simulink model "PubIfDecisionTOS_MDL"  (R2020b)
settings: configuration reference "DspaceConfig" (kept outside this file)
PostLoadFcn:
  | if any(exist('dsrtsu_mdlpostloadfcn', 'file') ~= 0), dsrtsu_mdlpostloadfcn('Execute', bdroot); end
InitFcn:
  | , if any(exist('dsmpb_private', 'file') ~= 0), dsmpb_private('dsmpb_mdlclblib', 'Init', bdroot); end,
undefined symbols (not defined in the file or in its folder): C_TOS_ACCEgoRAxletoFbumplength_m, C_TOS_ACCTargetFront_Flag, C_TOS_AEBJAPedObjDxThre_Val, C_TOS_AEBJAPedObjDyThre_Val, C_TOS_AEBJATargetSize_Val, C_TOS_AEBJAVehObjDxThre_Val, C_TOS_AEBJAVehObjDyThre_Val, C_TOS_AEBJuncPedTargetSize_Val, C_TOS_AEBLatObjDxThre_Val, C_TOS_AEBLatPedDyThre_Val, C_TOS_AEBLatTargetSize_Val, C_TOS_AEBLongTargetInEgoFront_Flag, C_TOS_axAbsGround_Parameter, C_TOS_CameraConfirmedFlag, C_TOS_CNsubjWidth, C_TOS_CurrentLaneCoreMinWidth_Val, C_TOS_CutInProb_Val_Zero, C_TOS_CutOutProb_Val_Zero, C_TOS_D2R_Val, C_TOS_DefaultValueObjectToCenterLine_dy, C_TOS_EgoCarWidth_Val, C_TOS_EgoDxRefPoint_m, C_TOS_EgoRAxletoFbumplength_m, C_TOS_HalfWidthVehicle_Con, C_TOS_HWA_CurrentLaneFlag, C_TOS_HWA_LeftLaneFlag, C_TOS_HWA_MovingDir_Vaild, C_TOS_HWA_MovState_Vaild, C_TOS_HWA_RightLaneFlag, C_TOS_LaneLineCourseErrorFront, C_TOS_LaneLineCourseErrorRear, C_TOS_MotorbikeDefaultWidth_m, C_TOS_NumberOfEffectiveTargets, C_TOS_Obj_Age_Val, C_TOS_Objdx_Constraint_Val, C_TOS_ObjectDefaultWidth_m, C_TOS_ObjInCurrentLane_Val, C_TOS_ObjInCurrentLaneValid, C_TOS_ObjInLeftLaneValid, C_TOS_ObjInRightLaneValid, C_TOS_ObjNotInCurrentLane_Val, C_TOS_ObjNotREElementType, C_TOS_ObjPredictDis_dy_ConstantVal_Zeros, C_TOS_ObjToCenterLine_ConstantVal_Zeros, C_TOS_OFMObjIDInvilad_Val, C_TOS_PIL_LatDisCons_Val_zero, C_TOS_PIL_ObjectCutInFlag_b, C_TOS_PIL_ObjectCutOutFlag_b, C_TOS_PIL_ObjLaneProb_al_Val, C_TOS_PP_ObjFusType_FC_Confirm_b, C_TOS_PP_ObjFusType_FC_FR_Confirm_b, C_TOS_PP_ObjFusType_FR_Confirm_b, C_TOS_RE_80BoolDefault_Val, C_TOS_RE_80Single181Default_Val, C_TOS_RE_80Single255Default_Val, C_TOS_RE_80Uint8Default_Val, C_TOS_RE_D2R, C_TOS_RE_D_180_Val, C_TOS_RE_InvalidObjectID_Val, C_TOS_RE_InvalidTargetChainDir_Val ... (+142)
libraries: simulink x1650, TOS_LIB x361, canfdmsglib x14
(part 24 of 69)

== system PubIfDecisionTOS_MDL/TOS_20201112/TOS_2012080320/PIL_1029/ObjCutInOut_Prob/ObjectCutOut/CutOutProb_Calculate/CutOutProb_Calculate/CutOutPredictDis_dy ==
  note: dx 修正vyc的 cut out 预测时间
  note: vyc的 cut out 基础预测时间
  ObjectToCenterLine_dy_Filt : Inport  OutDataTypeStr=single
  ObjectToCenterLine_dy : Inport  Port=2  OutDataTypeStr=single
  ObjectType : Inport  Port=3
  Object_DX : Inport  Port=4
  PP_ObjectToCenterLine_vyc : Inport  Port=5
  Object_VY : Inport  Port=6
  CutOutPredictTime : Subsystem
  CutOutPredictTime_Constraint1 : Subsystem
  CutOutPredictTime_Constraint2 : Subsystem
  PIL_CutOutPredictTime_ObserVale : Outport  OutDataTypeStr=single
  PIL_CutOutPredictTime_dxConstraint_ObserVale : Outport  Port=2  OutDataTypeStr=single
  CutOutPredictDis_dy : Outport  Port=3  OutDataTypeStr=single
  wires:
  Object_VY/1 -> CutOutPredictTime_Constraint2/4(Object_VY)
  Object_DX/1 -> CutOutPredictTime_Constraint1/2(Object_DX), CutOutPredictTime/5(Object_DX)
  ObjectToCenterLine_dy_Filt/1 -> CutOutPredictTime/1(ObjectToCenterLine_dy_Filt)
  ObjectToCenterLine_dy/1 -> [ObjectToCenterLine_dy], CutOutPredictTime/2(ObjectToCenterLin e_dy)
  CutOutPredictTime/1(CutOutPredictTime) -> [PIL_CutOutPredictTime_ObserVale], CutOutPredictTime_Constraint1/1(CutOutPredictTime)
  CutOutPredictTime_Constraint1/1(CutOutPredictTime_Constraint1) -> CutOutPredictTime_Constraint2/2(PredictTimeConstraint), [PIL_CutOutPredictTime_Constraint_ObserVale]
  PP_ObjectToCenterLine_vyc/1 -> CutOutPredictTime_Constraint2/3(PP_ObjectToCenterLine_vyc), [PP_ObjectToCenterLine_vyc]
  CutOutPredictTime_Constraint2/1(CutOutPredictDis_dy) -> CutOutPredictDis_dy/1
  [ObjectToCenterLine_dy] -> CutOutPredictTime_Constraint2/1(ObjectToCenterLine_dy)
  ObjectType/1 -> CutOutPredictTime/3(ObjectType)
  [PP_ObjectToCenterLine_vyc] -> CutOutPredictTime/4(PP_ObjectToCenterLine_vyc)
  [PIL_CutOutPredictTime_ObserVale] -> PIL_CutOutPredictTime_ObserVale/1
  [PIL_CutOutPredictTime_Constraint_ObserVale] -> PIL_CutOutPredictTime_dxConstraint_ObserVale/1

== system PubIfDecisionTOS_MDL/TOS_20201112/TOS_2012080320/PIL_1029/ObjCutInOut_Prob/ObjectCutOut/CutOutProb_Calculate/CutOutProb_Calculate/CutOutProb ==
  CutOutPredictDis_dy : Inport  OutDataTypeStr=single
  PIL_ObjectToCenterLine_dy_Filt : Inport  Port=2  OutDataTypeStr=single
  Object_Width : Inport  Port=3
  ObjectType : Inport  Port=4
  CutOutObjWidthConstraint : Subsystem
  CutOutProb_Calculation : Subsystem
  PIL_CutOutPredictDis_dy_ObjWidthConstraint_ObserVale : Outport
  CutOutProb : Outport  Port=2
  wires:
  ObjectType/1 -> CutOutObjWidthConstraint/4(ObjectType)
  CutOutProb_Calculation/1(CutOutProb_Calculation) -> CutOutProb/1  "CutInProb_ScopeConstraint"
  CutOutPredictDis_dy/1 -> CutOutObjWidthConstraint/1(CutOutPredictDis_dy)
  PIL_ObjectToCenterLine_dy_Filt/1 -> CutOutObjWidthConstraint/2(PIL_ObjectToCenterLine_dy_Filt), [ObjectToCenterLine_dy]
  Object_Width/1 -> CutOutObjWidthConstraint/3(Object_Width)
  CutOutObjWidthConstraint/1(CutOutPredictDis_dy_ObjWidthConstraint) -> [PIL_CutOutPredictDis_dy_ObjWidthConstraint_ObserVale], CutOutProb_Calculation/1(CutOutPredictDis_dy_ObjWidthConstraint)
  [ObjectToCenterLine_dy] -> CutOutProb_Calculation/2(PIL_ObjectToCenterLine_dy_Filt)
  [PIL_CutOutPredictDis_dy_ObjWidthConstraint_ObserVale] -> PIL_CutOutPredictDis_dy_ObjWidthConstraint_ObserVale/1

== system PubIfDecisionTOS_MDL/TOS_20201112/TOS_2012080320/PIL_1029/ObjCutInOut_Prob/ObjectCutOut/CutOutProb_Calculate/CutOutProb_Calculate/CutOutProb_ScopeConstraint ==
  note: cut out 计算概率值约束
  CutOutProb : Inport  OutDataTypeStr=single
  PIL_ObjectToCenterLine_dy_Filt : Inport  Port=2
  PP_ObjectToCenterLine_vyc : Inport  Port=3  OutDataTypeStr=single
  PP_ObjectToCenterLine_dy : Inport  Port=4  OutDataTypeStr=single
  Object_Width : Inport  Port=5
  ObjectType : Inport  Port=6
  C_CutInProb_Val_Zero : Constant  Value=C_TOS_CutOutProb_Val_Zero  OutDataTypeStr=single
      settings: AttributesFormatString=C_TOS_CutOutProb_Val_Zero = 0
  ObjectCutoutMind : Subsystem
  Switch : Switch  Criteria=u2 ~= 0  OutDataTypeStr=single
  PIL_ObjectCutOutMindFlg_ObserVale : Outport  OutDataTypeStr=boolean
  CutOutProb_ScopeConstraint : Outport  Port=2  OutDataTypeStr=single
  PIL_ObjectCutoutMindFlg1_ObserVale : Outport  Port=3  OutDataTypeStr=boolean
  PIL_ObjectCutoutMindFlg2_ObserVale : Outport  Port=4  OutDataTypeStr=boolean
  PIL_ObjectCutoutMindFlg3_ObserVale : Outport  Port=5  OutDataTypeStr=boolean
  wires:
  ObjectType/1 -> ObjectCutoutMind/5(ObjectType)
  PIL_ObjectToCenterLine_dy_Filt/1 -> ObjectCutoutMind/1(PIL_ObjectToCenterLine_dy_Filt)
  PP_ObjectToCenterLine_vyc/1 -> ObjectCutoutMind/2(PP_ObjectToCenterLine_vyc)
  C_CutInProb_Val_Zero/1 -> Switch/1
  CutOutProb/1 -> Switch/3
  Switch/1 -> CutOutProb_ScopeConstraint/1
  ObjectCutoutMind/1(ObjectCutoutMindFlg) -> [PIL_ObjectCutOutMindFlg_ObserVale], Switch/2
  PP_ObjectToCenterLine_dy/1 -> ObjectCutoutMind/3(PP_ObjectToCenterLine_dy)
  Object_Width/1 -> ObjectCutoutMind/4(Object_Width)
  [PIL_ObjectCutOutMindFlg_ObserVale] -> PIL_ObjectCutOutMindFlg_ObserVale/1
  ObjectCutoutMind/2(ObjectCutoutMindFlg1) -> [ObjectCutoutMindFlg1]
  ObjectCutoutMind/3(ObjectCutoutMindFlg2) -> [ObjectCutoutMindFlg2]
  ObjectCutoutMind/4(ObjectCutoutMindFlg3) -> [ObjectCutoutMindFlg3]
  [ObjectCutoutMindFlg1] -> PIL_ObjectCutoutMindFlg1_ObserVale/1
  [ObjectCutoutMindFlg2] -> PIL_ObjectCutoutMindFlg2_ObserVale/1
  [ObjectCutoutMindFlg3] -> PIL_ObjectCutoutMindFlg3_ObserVale/1

== system PubIfDecisionTOS_MDL/TOS_20201112/TOS_2012080320/PIL_1029/ProbCalculat/ProbCalculat/ObjectProbCalculation/ProbCalculation/LeftLane_LeftPro ==
  PIL_LeftCenterLine_dyc : Inport
  LeftLane_CoreArea_Boundary : Inport  Port=2
  LeftLane_EdgeLeft_Boundary : Inport  Port=3
  Constant1 : Constant  Value=C_TOS_ObjInCurrentLane_Val  OutDataTypeStr=single
      settings: AttributesFormatString=C_TOS_ObjInCurrentLane_Val = 1
  Constant2 : Constant  Value=C_TOS_PIL_LatDisCons_Val_zero
      settings: AttributesFormatString=C_TOS_PIL_LatDisCons_Val_zero = 0
  Constant3 : Constant  Value=C_TOS_ObjNotInCurrentLane_Val  OutDataTypeStr=single
      settings: AttributesFormatString=C_TOS_ObjNotInCurrentLane_Val = 0
  Divide3 : Product  Inputs=*/  OutDataTypeStr=single
  Min : MinMax  Function=max  Inputs=2
  Relational Operator1 : RelationalOperator  Operator=<  OutDataTypeStr=boolean  RndMeth=Nearest
  Relational Operator3 : RelationalOperator  Operator=>  OutDataTypeStr=boolean  RndMeth=Nearest
  Saturation : Saturate  UpperLimit=255  LowerLimit=0.001
  Subtract3 : Sum  Inputs=+-  OutDataTypeStr=single
  Subtract4 : Sum  Inputs=+-  OutDataTypeStr=single
  Switch1 : Switch  Criteria=u2 ~= 0  OutDataTypeStr=single
  Switch2 : Switch  Criteria=u2 ~= 0  OutDataTypeStr=single
  LeftLane_LeftPro : Outport
  wires:
  Divide3/1 -> Switch1/3
  Subtract4/1 -> Saturation/1
  Constant2/1 -> Min/1
  PIL_LeftCenterLine_dyc/1 -> Min/2
  [LeftLane_EdgeLeft_Boundary] -> Subtract4/1, Subtract3/1
  [LeftLane_CoreArea_Boundary] -> Subtract4/2
  Subtract3/1 -> Divide3/1
  [PIL_LeftCenterLine_dyc] -> Subtract3/2
  Switch2/1 -> LeftLane_LeftPro/1
  Switch1/1 -> Switch2/3
  Constant1/1 -> Switch1/1
  Relational Operator1/1 -> Switch1/2
  LeftLane_CoreArea_Boundary/1 -> [LeftLane_CoreArea_Boundary], Relational Operator1/2
  Constant3/1 -> Switch2/1
  Relational Operator3/1 -> Switch2/2
  LeftLane_EdgeLeft_Boundary/1 -> [LeftLane_EdgeLeft_Boundary], Relational Operator3/2
  Min/1 -> Relational Operator1/1, Relational Operator3/1, [PIL_LeftCenterLine_dyc]
  Saturation/1 -> Divide3/2

== system PubIfDecisionTOS_MDL/TOS_20201112/TOS_2012080320/PIL_1029/ProbCalculat/ProbCalculat/ObjectProbCalculation/ProbCalculation/LeftLane_RightPro ==
  PIL_LeftCenterLine_dyc : Inport
  LeftLane_CoreArea_Boundary : Inport  Port=2
  LeftLane_EdgeRight_Boundary : Inport  Port=3
  Abs : Abs
  Constant1 : Constant  Value=C_TOS_ObjInCurrentLane_Val  OutDataTypeStr=single
      settings: AttributesFormatString=C_TOS_ObjInCurrentLane_Val = 1
  Constant2 : Constant  Value=C_TOS_PIL_LatDisCons_Val_zero
      settings: AttributesFormatString=C_TOS_PIL_LatDisCons_Val_zero = 0
  Constant3 : Constant  Value=C_TOS_ObjNotInCurrentLane_Val  OutDataTypeStr=single
      settings: AttributesFormatString=C_TOS_ObjNotInCurrentLane_Val = 0
  Divide3 : Product  Inputs=*/  OutDataTypeStr=single
  Min : MinMax  Inputs=2
  Relational Operator1 : RelationalOperator  Operator=<  OutDataTypeStr=boolean  RndMeth=Nearest
  Relational Operator3 : RelationalOperator  Operator=>  OutDataTypeStr=boolean  RndMeth=Nearest
  Saturation : Saturate  UpperLimit=255  LowerLimit=0.001
  Subtract3 : Sum  Inputs=+-  OutDataTypeStr=single
  Subtract4 : Sum  Inputs=+-  OutDataTypeStr=single
  Switch1 : Switch  Criteria=u2 ~= 0  OutDataTypeStr=single
  Switch2 : Switch  Criteria=u2 ~= 0  OutDataTypeStr=single
  LeftLane_RightPro : Outport
  wires:
  Abs/1 -> [PIL_LeftCenterLine_dyc], Relational Operator3/1, Relational Operator1/1
  Saturation/1 -> Divide3/2
  Min/1 -> Abs/1
  LeftLane_EdgeRight_Boundary/1 -> Relational Operator3/2, [LeftLane_EdgeRight_Boundary]
  Relational Operator3/1 -> Switch2/2
  Constant3/1 -> Switch2/1
  LeftLane_CoreArea_Boundary/1 -> Relational Operator1/2, [LeftLane_CoreArea_Boundary]
  Relational Operator1/1 -> Switch1/2
  Constant1/1 -> Switch1/1
  Switch1/1 -> Switch2/3
  Switch2/1 -> LeftLane_RightPro/1
  [PIL_LeftCenterLine_dyc] -> Subtract3/2
  Subtract3/1 -> Divide3/1
  [LeftLane_CoreArea_Boundary] -> Subtract4/2
  [LeftLane_EdgeRight_Boundary] -> Subtract3/1, Subtract4/1
  PIL_LeftCenterLine_dyc/1 -> Min/2
  Constant2/1 -> Min/1
  Subtract4/1 -> Saturation/1
  Divide3/1 -> Switch1/3

== system PubIfDecisionTOS_MDL/TOS_20201112/TOS_2012080320/PIL_1029/ProbCalculat/ProbCalculat/ObjectProbCalculation/ProbCalculation/RightLane_LeftPro ==
  PIL_RightCenterLine_dyc : Inport
  RightLane_CoreArea_Boundary : Inport  Port=2
  RightLane_EdgeLeft_Boundary : Inport  Port=3
  Constant1 : Constant  Value=C_TOS_ObjInCurrentLane_Val  OutDataTypeStr=single
      settings: AttributesFormatString=C_TOS_ObjInCurrentLane_Val = 1
  Constant2 : Constant  Value=C_TOS_PIL_LatDisCons_Val_zero
      settings: AttributesFormatString=C_TOS_PIL_LatDisCons_Val_zero = 0
  Constant3 : Constant  Value=C_TOS_ObjNotInCurrentLane_Val  OutDataTypeStr=single
      settings: AttributesFormatString=C_TOS_ObjNotInCurrentLane_Val = 0
  Divide3 : Product  Inputs=*/  OutDataTypeStr=single
  Min : MinMax  Function=max  Inputs=2
  Relational Operator1 : RelationalOperator  Operator=<  OutDataTypeStr=boolean  RndMeth=Nearest
  Relational Operator3 : RelationalOperator  Operator=>  OutDataTypeStr=boolean  RndMeth=Nearest
  Saturation : Saturate  UpperLimit=255  LowerLimit=0.001
  Subtract3 : Sum  Inputs=+-  OutDataTypeStr=single
  Subtract4 : Sum  Inputs=+-  OutDataTypeStr=single
  Switch1 : Switch  Criteria=u2 ~= 0  OutDataTypeStr=single
  Switch2 : Switch  Criteria=u2 ~= 0  OutDataTypeStr=single
  RightLane_LeftPro : Outport
  wires:
  Saturation/1 -> Divide3/2
  Min/1 -> [PIL_RightCenterLine_dyc], Relational Operator3/1, Relational Operator1/1
  RightLane_EdgeLeft_Boundary/1 -> Relational Operator3/2, [RightLane_EdgeLeft_Boundary]
  Relational Operator3/1 -> Switch2/2
  Constant3/1 -> Switch2/1
  RightLane_CoreArea_Boundary/1 -> Relational Operator1/2, [RightLane_CoreArea_Boundary]
  Relational Operator1/1 -> Switch1/2
  Constant1/1 -> Switch1/1
  Switch1/1 -> Switch2/3
  Switch2/1 -> RightLane_LeftPro/1
  [PIL_RightCenterLine_dyc] -> Subtract3/2
  Subtract3/1 -> Divide3/1
  [RightLane_CoreArea_Boundary] -> Subtract4/2
  [RightLane_EdgeLeft_Boundary] -> Subtract3/1, Subtract4/1
  PIL_RightCenterLine_dyc/1 -> Min/2
  Constant2/1 -> Min/1
  Subtract4/1 -> Saturation/1
  Divide3/1 -> Switch1/3

== system PubIfDecisionTOS_MDL/TOS_20201112/TOS_2012080320/PIL_1029/ProbCalculat/ProbCalculat/ObjectProbCalculation/ProbCalculation/RightLane_RightPro ==
  PIL_RightCenterLine_dyc : Inport
  RightLane_CoreArea_Boundary : Inport  Port=2
  RightLane_EdgeRight_Boundary : Inport  Port=3
  Abs : Abs
  Constant1 : Constant  Value=C_TOS_ObjInCurrentLane_Val  OutDataTypeStr=single
      settings: AttributesFormatString=C_TOS_ObjInCurrentLane_Val = 1
  Constant2 : Constant  Value=C_TOS_PIL_LatDisCons_Val_zero
      settings: AttributesFormatString=C_TOS_PIL_LatDisCons_Val_zero = 0
  Constant3 : Constant  Value=C_TOS_ObjNotInCurrentLane_Val  OutDataTypeStr=single
      settings: AttributesFormatString=C_TOS_ObjNotInCurrentLane_Val = 0
  Divide3 : Product  Inputs=*/  OutDataTypeStr=single
  Min : MinMax  Inputs=2
  Relational Operator1 : RelationalOperator  Operator=<  OutDataTypeStr=boolean  RndMeth=Nearest
  Relational Operator3 : RelationalOperator  Operator=>  OutDataTypeStr=boolean  RndMeth=Nearest
  Saturation : Saturate  UpperLimit=255  LowerLimit=0.001
  Subtract3 : Sum  Inputs=+-  OutDataTypeStr=single
  Subtract4 : Sum  Inputs=+-  OutDataTypeStr=single
  Switch1 : Switch  Criteria=u2 ~= 0  OutDataTypeStr=single
  Switch2 : Switch  Criteria=u2 ~= 0  OutDataTypeStr=single
  RightLane_RightPro : Outport
  wires:
  Abs/1 -> Relational Operator1/1, Relational Operator3/1, [PIL_RightCenterLine_dyc]
  Divide3/1 -> Switch1/3
  Subtract4/1 -> Saturation/1
  Constant2/1 -> Min/1
  PIL_RightCenterLine_dyc/1 -> Min/2
  [RightLane_EdgeRight_Boundary] -> Subtract4/1, Subtract3/1
  [RightLane_CoreArea_Boundary] -> Subtract4/2
  Subtract3/1 -> Divide3/1
  [PIL_RightCenterLine_dyc] -> Subtract3/2
  Switch2/1 -> RightLane_RightPro/1
  Switch1/1 -> Switch2/3
  Constant1/1 -> Switch1/1
  Relational Operator1/1 -> Switch1/2
  RightLane_CoreArea_Boundary/1 -> [RightLane_CoreArea_Boundary], Relational Operator1/2
  Constant3/1 -> Switch2/1
  Relational Operator3/1 -> Switch2/2
  RightLane_EdgeRight_Boundary/1 -> [RightLane_EdgeRight_Boundary], Relational Operator3/2
  Min/1 -> Abs/1
  Saturation/1 -> Divide3/2

== system PubIfDecisionTOS_MDL/TOS_20201112/TOS_2012080320/PIL_1029/ProbCalculat/ProbCalculat/ObjectProbCalculation/ProbCalculation/SameLane_LeftPro ==
  PIL_SameCenterLine_dyc : Inport
  SameLane_CoreArea_Boundary : Inport  Port=2
  SameLane_EdgeLeft_Boundary : Inport  Port=3
  Constant : Constant  Commented=on  Value=P_TOS_CurrentLaneLeftBasicProb_Val  OutDataTypeStr=single
      settings: AttributesFormatString=P_TOS_CurrentLaneLeftBasicProb_Val = 0.5
  Constant1 : Constant  Value=C_TOS_ObjInCurrentLane_Val  OutDataTypeStr=single
      settings: AttributesFormatString=C_TOS_ObjInCurrentLane_Val = 1
  Constant2 : Constant  Value=C_TOS_PIL_LatDisCons_Val_zero
      settings: AttributesFormatString=C_TOS_PIL_LatDisCons_Val_zero = 0
  Constant3 : Constant  Value=C_TOS_ObjNotInCurrentLane_Val  OutDataTypeStr=single
      settings: AttributesFormatString=C_TOS_ObjNotInCurrentLane_Val = 0
  Divide3 : Product  Inputs=*/  OutDataTypeStr=single
  Min : MinMax  Function=max  Inputs=2
  Relational Operator1 : RelationalOperator  Operator=<  OutDataTypeStr=boolean  RndMeth=Nearest
  Relational Operator3 : RelationalOperator  Operator=>  OutDataTypeStr=boolean  RndMeth=Nearest
  Saturation : Saturate  UpperLimit=255  LowerLimit=0.001
  Subtract3 : Sum  Inputs=+-  OutDataTypeStr=single
  Subtract4 : Sum  Inputs=+-  OutDataTypeStr=single
  Switch1 : Switch  Criteria=u2 ~= 0  OutDataTypeStr=single
  Switch2 : Switch  Criteria=u2 ~= 0  OutDataTypeStr=single
  SameLane_LeftPro : Outport
  wires:
  Saturation/1 -> Divide3/2
  Min/1 -> [PIL_SameCenterLine_dyc], Relational Operator3/1, Relational Operator1/1
  SameLane_EdgeLeft_Boundary/1 -> Relational Operator3/2, [SameLane_EdgeLeft_Boundary]
  Relational Operator3/1 -> Switch2/2
  Constant3/1 -> Switch2/1
  SameLane_CoreArea_Boundary/1 -> Relational Operator1/2, [SameLane_CoreArea_Boundary]
  Relational Operator1/1 -> Switch1/2
  Constant1/1 -> Switch1/1
  Switch1/1 -> Switch2/3
  Switch2/1 -> SameLane_LeftPro/1
  [PIL_SameCenterLine_dyc] -> Subtract3/2
  Subtract3/1 -> Divide3/1
  [SameLane_CoreArea_Boundary] -> Subtract4/2
  [SameLane_EdgeLeft_Boundary] -> Subtract3/1, Subtract4/1
  PIL_SameCenterLine_dyc/1 -> Min/2
  Constant2/1 -> Min/1
  Subtract4/1 -> Saturation/1
  Divide3/1 -> Switch1/3

== system PubIfDecisionTOS_MDL/TOS_20201112/TOS_2012080320/PIL_1029/ProbCalculat/ProbCalculat/ObjectProbCalculation/ProbCalculation/SameLane_RightPro ==
  PIL_SameCenterLine_dyc : Inport
  SameLane_CoreArea_Boundary : Inport  Port=2
  SameLane_EdgeRight_Boundary : Inport  Port=3
  Abs : Abs
  Constant1 : Constant  Value=C_TOS_ObjInCurrentLane_Val  OutDataTypeStr=single
      settings: AttributesFormatString=C_TOS_ObjInCurrentLane_Val = 1
  Constant2 : Constant  Value=C_TOS_PIL_LatDisCons_Val_zero
      settings: AttributesFormatString=C_TOS_PIL_LatDisCons_Val_zero = 0
  Constant3 : Constant  Value=C_TOS_ObjNotInCurrentLane_Val  OutDataTypeStr=single
      settings: AttributesFormatString=C_TOS_ObjNotInCurrentLane_Val = 0
  Constant4 : Constant  Commented=on  Value=P_TOS_CurrentLaneRightBasicProb_Val  OutDataTypeStr=single
      settings: AttributesFormatString=P_TOS_CurrentLaneRightBasicProb_Val = 0.5
  Divide3 : Product  Inputs=*/  OutDataTypeStr=single
  Min : MinMax  Inputs=2
  Relational Operator1 : RelationalOperator  Operator=<  OutDataTypeStr=boolean  RndMeth=Nearest
  Relational Operator3 : RelationalOperator  Operator=>  OutDataTypeStr=boolean  RndMeth=Nearest
  Saturation : Saturate  UpperLimit=255  LowerLimit=0.001
  Subtract3 : Sum  Inputs=+-  OutDataTypeStr=single
  Subtract4 : Sum  Inputs=+-  OutDataTypeStr=single
  Switch1 : Switch  Criteria=u2 ~= 0  OutDataTypeStr=single
  Switch2 : Switch  Criteria=u2 ~= 0  OutDataTypeStr=single
  SameLane_RightPro : Outport
  wires:
  Abs/1 -> Relational Operator1/1, Relational Operator3/1, [PIL_SameCenterLine_dyc]
  Divide3/1 -> Switch1/3
  Subtract4/1 -> Saturation/1
  Constant2/1 -> Min/1
  PIL_SameCenterLine_dyc/1 -> Min/2
  [SameLane_EdgeRight_Boundary] -> Subtract4/1, Subtract3/1
  [SameLane_CoreArea_Boundary] -> Subtract4/2
  Subtract3/1 -> Divide3/1
  [PIL_SameCenterLine_dyc] -> Subtract3/2
  Switch2/1 -> SameLane_RightPro/1
  Switch1/1 -> Switch2/3
  Constant1/1 -> Switch1/1
  Relational Operator1/1 -> Switch1/2
  SameLane_CoreArea_Boundary/1 -> [SameLane_CoreArea_Boundary], Relational Operator1/2
  Constant3/1 -> Switch2/1
  Relational Operator3/1 -> Switch2/2
  SameLane_EdgeRight_Boundary/1 -> [SameLane_EdgeRight_Boundary], Relational Operator3/2
  Min/1 -> Abs/1
  Saturation/1 -> Divide3/2

== system PubIfDecisionTOS_MDL/TOS_20201112/TOS_2012080320/PIL_1029/ProbCalculat/ProbCalculat/Subsystem/EgoVehiclePro/EgoLaneProb ==
  HalfEgoWidth : Inport
  t_dleft_EgoLane : Inport  Port=2
  t_dright_EgoLane : Inport  Port=3
  Add : Sum  Inputs=+-
  Add1 : Sum  Inputs=+-
  Add2 : Sum  Inputs=+-
  Constant : Constant  Value=0  OutDataTypeStr=single
  Constant1 : Constant  OutDataTypeStr=single
  Constant2 : Constant  Value=0  OutDataTypeStr=single
  Constant3 : Constant  OutDataTypeStr=single
  Divide : Product  Inputs=*/
  Divide1 : Product  Inputs=*/
  Gain1 : Gain  Gain=-1
  Gain2 : Gain  Gain=2
  Gain3 : Gain  Gain=-1
  Gain4 : Gain  Gain=2
  Relational Operator1 : RelationalOperator  Operator=<=  OutDataTypeStr=boolean  RndMeth=Nearest
  Relational Operator2 : RelationalOperator  Operator=>  OutDataTypeStr=boolean  RndMeth=Nearest
  Relational Operator3 : RelationalOperator  Operator=<=  OutDataTypeStr=boolean  RndMeth=Nearest
  Relational Operator4 : RelationalOperator  Operator=>  OutDataTypeStr=boolean  RndMeth=Nearest
  Switch{1..4} (4 alike) : Switch  Criteria=u2 > Threshold
  " EgoLaneProb" : Outport
  wires:
  Switch2/1 -> Add2/1  "t_dleftProb"
  t_dleft_EgoLane/1 -> Add/1, Relational Operator2/1, Relational Operator1/1
  Gain1/1 -> Relational Operator1/2, Add/2
  Relational Operator1/1 -> Switch2/2
  Constant/1 -> Switch2/1
  Relational Operator2/1 -> Switch1/2
  Switch1/1 -> Switch2/3
  Constant1/1 -> Switch1/1
  Add/1 -> Divide/1
  Divide/1 -> Switch1/3
  Gain2/1 -> Divide/2
  Gain4/1 -> Divide1/2
  HalfEgoWidth/1 -> Gain2/1, Gain3/1, Relational Operator4/2, Gain4/1, Relational Operator2/2, Gain1/1
  Divide1/1 -> Switch3/3
  Add1/1 -> Divide1/1
  Constant3/1 -> Switch3/1
  Switch3/1 -> Switch4/3
  Relational Operator4/1 -> Switch3/2
  Constant2/1 -> Switch4/1
  Relational Operator3/1 -> Switch4/2
  Gain3/1 -> Add1/2, Relational Operator3/2
  t_dright_EgoLane/1 -> Relational Operator3/1, Relational Operator4/1, Add1/1
  Switch4/1 -> Add2/2  "t_drightProb"
  Add2/1 -> " EgoLaneProb"/1

== system PubIfDecisionTOS_MDL/TOS_20201112/TOS_2012080320/PIL_1029/ProbCalculat/ProbCalculat/Subsystem/EgoVehiclePro/LeftLaneProb ==
  HalfEgoWidth : Inport
  t_dleft_LeftLane : Inport  Port=2
  t_dright_LeftLane : Inport  Port=3
  Add : Sum  Inputs=+-
  Add1 : Sum  Inputs=+-
  Add2 : Sum  Inputs=+-
  Constant : Constant  Value=0  OutDataTypeStr=single
  Constant1 : Constant  OutDataTypeStr=single
  Constant2 : Constant  Value=0  OutDataTypeStr=single
  Constant3 : Constant  OutDataTypeStr=single
  Divide : Product  Inputs=*/  OutDataTypeStr=single
  Divide1 : Product  Inputs=*/  OutDataTypeStr=single
  Gain1 : Gain  Gain=-1
  Gain2 : Gain  Gain=2
  Gain3 : Gain  Gain=-1
  Gain4 : Gain  Gain=2
  Relational Operator1 : RelationalOperator  Operator=<=  OutDataTypeStr=boolean  RndMeth=Nearest
  Relational Operator2 : RelationalOperator  Operator=>  OutDataTypeStr=boolean  RndMeth=Nearest
  Relational Operator3 : RelationalOperator  Operator=<=  OutDataTypeStr=boolean  RndMeth=Nearest
  Relational Operator4 : RelationalOperator  Operator=>  OutDataTypeStr=boolean  RndMeth=Nearest
  Switch{1..4} (4 alike) : Switch  Criteria=u2 > Threshold
  " LeftLaneProb" : Outport
  wires:
  Switch4/1 -> Add2/2  "t_drightProb"
  t_dright_LeftLane/1 -> Add1/1, Relational Operator4/1, Relational Operator3/1
  Gain3/1 -> Relational Operator3/2, Add1/2
  Relational Operator3/1 -> Switch4/2
  Constant2/1 -> Switch4/1
  Relational Operator4/1 -> Switch3/2
  Switch3/1 -> Switch4/3
  Constant3/1 -> Switch3/1
  Add1/1 -> Divide1/1
  Divide1/1 -> Switch3/3
  HalfEgoWidth/1 -> Gain1/1, Relational Operator2/2, Gain4/1, Relational Operator4/2, Gain3/1, Gain2/1
  Gain4/1 -> Divide1/2
  Gain2/1 -> Divide/2
  Divide/1 -> Switch1/3
  Add/1 -> Divide/1
  Constant1/1 -> Switch1/1
  Switch1/1 -> Switch2/3
  Relational Operator2/1 -> Switch1/2
  Constant/1 -> Switch2/1
  Relational Operator1/1 -> Switch2/2
  Gain1/1 -> Add/2, Relational Operator1/2
  t_dleft_LeftLane/1 -> Relational Operator1/1, Relational Operator2/1, Add/1
  Switch2/1 -> Add2/1  "t_dleftProb"
  Add2/1 -> " LeftLaneProb"/1

== system PubIfDecisionTOS_MDL/TOS_20201112/TOS_2012080320/PIL_1029/ProbCalculat/ProbCalculat/Subsystem/EgoVehiclePro/RightLaneProb ==
  HalfEgoWidth : Inport
  t_dleft_RightLane : Inport  Port=2
  t_dright_RightLane : Inport  Port=3
  Add : Sum  Inputs=+-
  Add1 : Sum  Inputs=+-
  Add2 : Sum  Inputs=+-
  Constant : Constant  Value=0  OutDataTypeStr=single
  Constant1 : Constant  OutDataTypeStr=single
  Constant2 : Constant  Value=0  OutDataTypeStr=single
  Constant3 : Constant  OutDataTypeStr=single
  Divide : Product  Inputs=*/
  Divide1 : Product  Inputs=*/
  Gain1 : Gain  Gain=-1
  Gain2 : Gain  Gain=2
  Gain3 : Gain  Gain=-1
  Gain4 : Gain  Gain=2
  Relational Operator1 : RelationalOperator  Operator=<=  OutDataTypeStr=boolean  RndMeth=Nearest
  Relational Operator2 : RelationalOperator  Operator=>  OutDataTypeStr=boolean  RndMeth=Nearest
  Relational Operator3 : RelationalOperator  Operator=<=  OutDataTypeStr=boolean  RndMeth=Nearest
  Relational Operator4 : RelationalOperator  Operator=>  OutDataTypeStr=boolean  RndMeth=Nearest
  Switch{1..4} (4 alike) : Switch  Criteria=u2 > Threshold
  " RightLaneProb" : Outport
  wires:
  t_dleft_RightLane/1 -> Add/1, Relational Operator2/1, Relational Operator1/1
  Gain1/1 -> Relational Operator1/2, Add/2
  Relational Operator1/1 -> Switch2/2
  Constant/1 -> Switch2/1
  Relational Operator2/1 -> Switch1/2
  Switch1/1 -> Switch2/3
  Constant1/1 -> Switch1/1
  Add/1 -> Divide/1
  Divide/1 -> Switch1/3
  Gain2/1 -> Divide/2
  Gain4/1 -> Divide1/2
  HalfEgoWidth/1 -> Gain2/1, Gain3/1, Relational Operator4/2, Gain4/1, Relational Operator2/2, Gain1/1
  Divide1/1 -> Switch3/3
  Add1/1 -> Divide1/1
  Constant3/1 -> Switch3/1
  Switch3/1 -> Switch4/3
  Relational Operator4/1 -> Switch3/2
  Constant2/1 -> Switch4/1
  Relational Operator3/1 -> Switch4/2
  Gain3/1 -> Add1/2, Relational Operator3/2
  t_dright_RightLane/1 -> Relational Operator3/1, Relational Operator4/1, Add1/1
  Add2/1 -> " RightLaneProb"/1
  Switch2/1 -> Add2/1  "t_dleftProb"
  Switch4/1 -> Add2/2  "t_drightProb"

== system PubIfDecisionTOS_MDL/TOS_20201112/TOS_2012080320/PIL_1029/ProbCalculat/ProbCalculat/Subsystem/PIL_EgoVehiclePro/EgoVehicle_EgoLaneProb ==
  EgoCar_CurrentLaneProb : Inport
  Add : Sum  Inputs=++++
  Add1 : Sum  Inputs=++++
  Bus Creator : BusCreator  Inputs=4
  Bus Selector : BusSelector  OutputSignals=Out_Prob1.Count1,Out_Prob2.Count2,Out_Prob3.Count3,Out_Prob4.Count4
  Bus Selector2 : BusSelector  OutputSignals=Out_Prob1.Prob1,Out_Prob2.Prob2,Out_Prob3.Prob3,Out_Prob4.Prob4
  Compare To Constant : simulink/Logic and Bit Operations/Compare To Constant  relop=~=  const=0  OutDataTypeStr=boolean
  Constant1 : Constant  OutDataTypeStr=single
  Data1 : Subsystem
  Data10 : Subsystem
  Data2 : Subsystem
  Data3 : Subsystem
  Data4 : Subsystem
  Data5 : Subsystem
  Data6 : Subsystem
  Data7 : Subsystem
  Data8 : Subsystem
  Data9 : Subsystem
  Delay : Delay  DelayLength=1  InitialCondition=0
  Delay1 : Delay  InitialCondition=0
  Delay2 : Delay  DelayLength=3  InitialCondition=0
  Delay3 : Delay  DelayLength=4  InitialCondition=0
  Delay4 : Delay  DelayLength=5  InitialCondition=0
  Delay5 : Delay  DelayLength=6  InitialCondition=0
  Delay6 : Delay  DelayLength=7  InitialCondition=0
  Delay7 : Delay  DelayLength=8  InitialCondition=0
  Delay8 : Delay  DelayLength=9  InitialCondition=0
  Divide : Product  Inputs=*/
  Switch : Switch  Criteria=u2 > Threshold
  Terminator{,1..5} (6 alike) : Terminator
  EgoCar_CurrentLaneProb_Filt : Outport
  wires:
  Switch/1 -> Divide/2
  Delay5/1 -> Data7/1(Prob)
  Delay3/1 -> Data5/1(Prob)
  Data4/1(Out_Prob4) -> Bus Creator/4
  Delay1/1 -> Data3/1(Prob)
  Delay8/1 -> Data10/1(Prob)
  Data8/1(Out_Prob8) -> Terminator3/1
  Add/1 -> Compare To Constant/1, Switch/1
  Constant1/1 -> Switch/3
  Delay6/1 -> Data8/1(Prob)
  Data10/1(Out_Prob10) -> Terminator5/1
  Compare To Constant/1 -> Switch/2
  Data5/1(Out_Prob5) -> Terminator/1
  Bus Creator/1 -> Bus Selector/1, Bus Selector2/1
  Data2/1(Out_Prob2) -> Bus Creator/2
  Data1/1(Out_Prob1) -> Bus Creator/1
  Data9/1(Out_Prob9) -> Terminator4/1
  Delay7/1 -> Data9/1(Prob)
  Delay4/1 -> Data6/1(Prob)
  Delay/1 -> Data2/1(Prob)
  Data6/1(Out_Prob6) -> Terminator1/1
  Data7/1(Out_Prob7) -> Terminator2/1
  Delay2/1 -> Data4/1(Prob)
  EgoCar_CurrentLaneProb/1 -> Delay1/1, Delay8/1, Delay7/1, Delay6/1, Delay5/1, Delay4/1, Delay3/1, Delay2/1, Delay/1, Data1/1(Prob)
  Add1/1 -> Divide/1
  Data3/1(Out_Prob3) -> Bus Creator/3
  Divide/1 -> EgoCar_CurrentLaneProb_Filt/1
  Bus Selector/1 -> Add/1  "<Count1>"
  Bus Selector/2 -> Add/2  "<Count2>"
  Bus Selector/3 -> Add/3  "<Count3>"
  Bus Selector/4 -> Add/4  "<Count4>"
  Bus Selector2/1 -> Add1/1  "<Prob1>"
  Bus Selector2/2 -> Add1/2  "<Prob2>"
  Bus Selector2/3 -> Add1/3  "<Prob3>"
  Bus Selector2/4 -> Add1/4  "<Prob4>"

== system PubIfDecisionTOS_MDL/TOS_20201112/TOS_2012080320/PIL_1029/ProbCalculat/ProbCalculat/Subsystem/PIL_EgoVehiclePro/EgoVehicle_LeftLaneProb ==
  EgoVehicle_LeftLaneProb : Inport
  Add : Sum  Inputs=++++
  Add1 : Sum  Inputs=++++
  Bus Creator : BusCreator  Inputs=4
  Bus Selector : BusSelector  OutputSignals=Out_Prob1.Count1,Out_Prob2.Count2,Out_Prob3.Count3,Out_Prob4.Count4
  Bus Selector2 : BusSelector  OutputSignals=Out_Prob1.Prob1,Out_Prob2.Prob2,Out_Prob3.Prob3,Out_Prob4.Prob4
  Compare To Constant : simulink/Logic and Bit Operations/Compare To Constant  relop=~=  const=0  OutDataTypeStr=boolean
  Constant1 : Constant  OutDataTypeStr=single
  Data1 : Subsystem
  Data10 : Subsystem
  Data2 : Subsystem
  Data3 : Subsystem
  Data4 : Subsystem
  Data5 : Subsystem
  Data6 : Subsystem
  Data7 : Subsystem
  Data8 : Subsystem
  Data9 : Subsystem
  Delay : Delay  DelayLength=1  InitialCondition=0
  Delay1 : Delay  InitialCondition=0
  Delay2 : Delay  DelayLength=3  InitialCondition=0
  Delay3 : Delay  DelayLength=4  InitialCondition=0
  Delay4 : Delay  DelayLength=5  InitialCondition=0
  Delay5 : Delay  DelayLength=6  InitialCondition=0
  Delay6 : Delay  DelayLength=7  InitialCondition=0
  Delay7 : Delay  DelayLength=8  InitialCondition=0
  Delay8 : Delay  DelayLength=9  InitialCondition=0
  Divide : Product  Inputs=*/
  Switch : Switch  Criteria=u2 > Threshold
  Terminator{,1..5} (6 alike) : Terminator
  EgoVehicle_LeftLaneProb_Filt : Outport
  wires:
  Divide/1 -> EgoVehicle_LeftLaneProb_Filt/1
  Data3/1(Out_Prob3) -> Bus Creator/3
  Add1/1 -> Divide/1
  EgoVehicle_LeftLaneProb/1 -> Data1/1(Prob), Delay/1, Delay2/1, Delay3/1, Delay4/1, Delay5/1, Delay6/1, Delay7/1, Delay8/1, Delay1/1
  Delay2/1 -> Data4/1(Prob)
  Data7/1(Out_Prob7) -> Terminator2/1
  Data6/1(Out_Prob6) -> Terminator1/1
  Delay/1 -> Data2/1(Prob)
  Delay4/1 -> Data6/1(Prob)
  Delay7/1 -> Data9/1(Prob)
  Data9/1(Out_Prob9) -> Terminator4/1
  Data1/1(Out_Prob1) -> Bus Creator/1
  Data2/1(Out_Prob2) -> Bus Creator/2
  Bus Creator/1 -> Bus Selector2/1, Bus Selector/1
  Data5/1(Out_Prob5) -> Terminator/1
  Compare To Constant/1 -> Switch/2
  Data10/1(Out_Prob10) -> Terminator5/1
  Bus Selector/1 -> Add/1  "<Count1>"
  Delay6/1 -> Data8/1(Prob)
  Constant1/1 -> Switch/3
  Add/1 -> Switch/1, Compare To Constant/1
  Data8/1(Out_Prob8) -> Terminator3/1
  Delay8/1 -> Data10/1(Prob)
  Delay1/1 -> Data3/1(Prob)
  Data4/1(Out_Prob4) -> Bus Creator/4
  Delay3/1 -> Data5/1(Prob)
  Delay5/1 -> Data7/1(Prob)
  Switch/1 -> Divide/2
  Bus Selector/2 -> Add/2  "<Count2>"
  Bus Selector/3 -> Add/3  "<Count3>"
  Bus Selector/4 -> Add/4  "<Count4>"
  Bus Selector2/1 -> Add1/1  "<Prob1>"
  Bus Selector2/2 -> Add1/2  "<Prob2>"
  Bus Selector2/3 -> Add1/3  "<Prob3>"
  Bus Selector2/4 -> Add1/4  "<Prob4>"

== system PubIfDecisionTOS_MDL/TOS_20201112/TOS_2012080320/PIL_1029/ProbCalculat/ProbCalculat/Subsystem/PIL_EgoVehiclePro/EgoVehicle_RightLaneProb ==
  EgoVehicle_RightLaneProb : Inport
  Add : Sum  Inputs=++++
  Add1 : Sum  Inputs=++++
  Bus Creator1 : BusCreator  Inputs=4
  Bus Selector : BusSelector  OutputSignals=Out_Prob1.Count1,Out_Prob2.Count2,Out_Prob3.Count3,Out_Prob4.Count4
  Bus Selector2 : BusSelector  OutputSignals=Out_Prob1.Prob1,Out_Prob2.Prob2,Out_Prob3.Prob3,Out_Prob4.Prob4
  Compare To Constant : simulink/Logic and Bit Operations/Compare To Constant  relop=~=  const=0  OutDataTypeStr=boolean
  Constant1 : Constant  OutDataTypeStr=single
  Data1 : Subsystem
  Data10 : Subsystem
  Data2 : Subsystem
  Data3 : Subsystem
  Data4 : Subsystem
  Data5 : Subsystem
  Data6 : Subsystem
  Data7 : Subsystem
  Data8 : Subsystem
  Data9 : Subsystem
  Delay : Delay  DelayLength=1  InitialCondition=0
  Delay1 : Delay  InitialCondition=0
  Delay2 : Delay  DelayLength=3  InitialCondition=0
  Delay3 : Delay  DelayLength=4  InitialCondition=0
  Delay4 : Delay  DelayLength=5  InitialCondition=0
  Delay5 : Delay  DelayLength=6  InitialCondition=0
  Delay6 : Delay  DelayLength=7  InitialCondition=0
  Delay7 : Delay  DelayLength=8  InitialCondition=0
  Delay8 : Delay  DelayLength=9  InitialCondition=0
  Divide : Product  Inputs=*/
  Switch : Switch  Criteria=u2 > Threshold
  Terminator{6..11} (6 alike) : Terminator
  EgoVehicle_RightLaneProb_Filt : Outport
  wires:
  Divide/1 -> EgoVehicle_RightLaneProb_Filt/1
  Data3/1(Out_Prob3) -> Bus Creator1/3
  Add1/1 -> Divide/1
  EgoVehicle_RightLaneProb/1 -> Data1/1(Prob), Delay/1, Delay2/1, Delay3/1, Delay4/1, Delay5/1, Delay6/1, Delay7/1, Delay8/1, Delay1/1
  Delay2/1 -> Data4/1(Prob)
  Data7/1(Out_Prob7) -> Terminator8/1
  Data6/1(Out_Prob6) -> Terminator7/1
  Delay/1 -> Data2/1(Prob)
  Delay4/1 -> Data6/1(Prob)
  Delay7/1 -> Data9/1(Prob)
  Data9/1(Out_Prob9) -> Terminator10/1
  Data1/1(Out_Prob1) -> Bus Creator1/1
  Data2/1(Out_Prob2) -> Bus Creator1/2
  Bus Creator1/1 -> Bus Selector2/1, Bus Selector/1
  Data5/1(Out_Prob5) -> Terminator6/1
  Compare To Constant/1 -> Switch/2
  Data10/1(Out_Prob10) -> Terminator11/1
  Delay6/1 -> Data8/1(Prob)
  Constant1/1 -> Switch/3
  Add/1 -> Switch/1, Compare To Constant/1
  Data8/1(Out_Prob8) -> Terminator9/1
  Delay8/1 -> Data10/1(Prob)
  Delay1/1 -> Data3/1(Prob)
  Data4/1(Out_Prob4) -> Bus Creator1/4
  Delay3/1 -> Data5/1(Prob)
  Delay5/1 -> Data7/1(Prob)
  Switch/1 -> Divide/2
  Bus Selector2/1 -> Add1/1  "<Prob1>"
  Bus Selector2/2 -> Add1/2  "<Prob2>"
  Bus Selector2/3 -> Add1/3  "<Prob3>"
  Bus Selector2/4 -> Add1/4  "<Prob4>"
  Bus Selector/1 -> Add/1  "<Count1>"
  Bus Selector/2 -> Add/2  "<Count2>"
  Bus Selector/3 -> Add/3  "<Count3>"
  Bus Selector/4 -> Add/4  "<Count4>"

== system PubIfDecisionTOS_MDL/TOS_20201112/TOS_2012080320/PP1128/AAT-AdditionalAttributes/PP_CenterLine_Calculat/LaneWidth_80/LaneWidth/PP_LaneWidth ==
  LM_SignalVerification : Inport
  Action Port : ActionPort
  Add : Sum  Inputs=+-  OutDataTypeStr=single
  Add1 : Sum  Inputs=+-  OutDataTypeStr=single
  Add2 : Sum  Inputs=+-  OutDataTypeStr=single
  Bus Selector : BusSelector  OutputSignals=LM_LL_pC0,LM_LR_pC0,LM_RL_pC0,LM_RR_pC0
  Saturation : Saturate  UpperLimit=4.5  LowerLimit=2.0  OutDataTypeStr=single
  Saturation1 : Saturate  UpperLimit=4.5  LowerLimit=2.0  OutDataTypeStr=single
  Saturation2 : Saturate  UpperLimit=4.5  LowerLimit=2.0  OutDataTypeStr=single
  Signal Copy{,1..3} (4 alike) : SignalConversion  OverrideOpt=off
  TOS_PP_LeftLaneWidth : Outport
  TOS_PP_CurrentLaneWidth : Outport  Port=2
  TOS_PP_RightLaneWidth : Outport  Port=3
  wires:
  Bus Selector/1 -> Signal Copy/1  "<LM_LL_pC0>"
  Bus Selector/4 -> Signal Copy3/1  "<LM_RR_pC0>"
  LM_SignalVerification/1 -> Bus Selector/1
  Bus Selector/3 -> Signal Copy2/1  "<LM_RL_pC0>"
  Bus Selector/2 -> Signal Copy1/1  "<LM_LR_pC0>"
  Add/1 -> Saturation/1
  Add2/1 -> Saturation2/1
  Add1/1 -> Saturation1/1
  Signal Copy1/1 -> Add/2, Add1/1  "LM_LR_pC0"
  Signal Copy/1 -> Add/1  "LM_LL_pC0"
  Signal Copy3/1 -> Add2/2  "LM_RR_pC0"
  Signal Copy2/1 -> Add2/1, Add1/2  "LM_RL_pC0"
  Saturation/1 -> TOS_PP_LeftLaneWidth/1
  Saturation1/1 -> TOS_PP_CurrentLaneWidth/1
  Saturation2/1 -> TOS_PP_RightLaneWidth/1

== system PubIfDecisionTOS_MDL/TOS_20201112/TOS_2012080320/PP1128/AAT-AdditionalAttributes/PP_CenterLine_Calculat/LaneWidth_80/LaneWidth/PP_LaneWidthDefalut ==
  Action Port : ActionPort
  Constant1 : Constant  Value=0  OutDataTypeStr=single
  Constant2 : Constant  Value=0  OutDataTypeStr=single
  Constant3 : Constant  Value=0  OutDataTypeStr=single
  TOS_PP_LeftLaneWidth : Outport
  TOS_PP_CurrentLaneWidth : Outport  Port=2
  TOS_PP_RightLaneWidth : Outport  Port=3
  wires:
  Constant3/1 -> TOS_PP_RightLaneWidth/1  "TOS_PP_RightLaneWidth"
  Constant1/1 -> TOS_PP_LeftLaneWidth/1  "TOS_PP_LeftLaneWidth"
  Constant2/1 -> TOS_PP_CurrentLaneWidth/1  "TOS_PP_CurrentLaneWidth"

== system PubIfDecisionTOS_MDL/TOS_20201112/TOS_2012080320/PP1128/AAT-AdditionalAttributes/PP_CenterLine_Calculat/LaneWidth_80/LaneWidth/PP_StaticObj_LaneWidth ==
  LM_SignalVerification : Inport
  Action Port : ActionPort
  Add : Sum  Inputs=+-  OutDataTypeStr=single
  Add1 : Sum  Inputs=+-  OutDataTypeStr=single
  Add2 : Sum  Inputs=+-  OutDataTypeStr=single
  Bus Selector : BusSelector  OutputSignals=LM_LL_pC0,LM_LR_pC0,LM_RL_pC0,LM_RR_pC0
  Constant3 : Constant  Value=2.4  OutDataTypeStr=single
  Max : MinMax  Inputs=2
  Max1 : MinMax  Inputs=2
  Max2 : MinMax  Inputs=2
  Saturation : Saturate  UpperLimit=4.5  LowerLimit=2.0  OutDataTypeStr=single
  Saturation1 : Saturate  UpperLimit=4.5  LowerLimit=2.0  OutDataTypeStr=single
  Saturation2 : Saturate  UpperLimit=4.5  LowerLimit=2.0  OutDataTypeStr=single
  Signal Copy{,1..3} (4 alike) : SignalConversion  OverrideOpt=off
  TOS_PP_LeftLaneWidth : Outport
  TOS_PP_CurrentLaneWidth : Outport  Port=2
  TOS_PP_RightLaneWidth : Outport  Port=3
  wires:
  Max2/1 -> TOS_PP_RightLaneWidth/1
  Constant3/1 -> Max/1, Max1/1, Max2/1
  Max1/1 -> TOS_PP_CurrentLaneWidth/1
  Max/1 -> TOS_PP_LeftLaneWidth/1
  Saturation2/1 -> Max2/2
  Saturation1/1 -> Max1/2
  Saturation/1 -> Max/2
  Signal Copy2/1 -> Add1/2, Add2/1  "LM_RL_pC0"
  Signal Copy3/1 -> Add2/2  "LM_RR_pC0"
  Signal Copy/1 -> Add/1  "LM_LL_pC0"
  Signal Copy1/1 -> Add1/1, Add/2  "LM_LR_pC0"
  Add1/1 -> Saturation1/1
  Add2/1 -> Saturation2/1
  Add/1 -> Saturation/1
  Bus Selector/2 -> Signal Copy1/1  "<LM_LR_pC0>"
  Bus Selector/3 -> Signal Copy2/1  "<LM_RL_pC0>"
  LM_SignalVerification/1 -> Bus Selector/1
  Bus Selector/4 -> Signal Copy3/1  "<LM_RR_pC0>"
  Bus Selector/1 -> Signal Copy/1  "<LM_LL_pC0>"

== system PubIfDecisionTOS_MDL/TOS_20201112/TOS_2012080320/PP1128/AAT-AdditionalAttributes/PP_ObjectToCenterLine_dy/PP_EgoVeh_Object_ToCenterLine/PP_ObjectToCenterLine/PP_ObjectToCenterLineDefault ==
  Action Port : ActionPort  ActionPortLabel=if(u1 ~= 0)
  Constant2 : Constant  Value=255  OutDataTypeStr=single
  PP_ObjectToCenterLine_dy : Outport
  wires:
  Constant2/1 -> PP_ObjectToCenterLine_dy/1

== system PubIfDecisionTOS_MDL/TOS_20201112/TOS_2012080320/PP1128/AAT-AdditionalAttributes/PP_ObjectToCenterLine_dy/PP_EgoVeh_Object_ToCenterLine/PP_ObjectToCenterLine/PP_ObjectToCenterLine_ ==
  Object_DY : Inport
  Object_DX : Inport  Port=2
  line01_C0 : Inport  Port=3
  line01_C1 : Inport  Port=4
  line01_C2 : Inport  Port=5
  line01_C3 : Inport  Port=6
  line01_dDisStart : Inport  Port=7
  line01_dDisEnd : Inport  Port=8
  line02_C0 : Inport  Port=9
  line02_C1 : Inport  Port=10
  line02_C2 : Inport  Port=11
  line02_C3 : Inport  Port=12
  line02_dDisStart : Inport  Port=13
  line02_dDisEnd : Inport  Port=14
  line03_C0 : Inport  Port=15
  line03_C1 : Inport  Port=16
  line03_C2 : Inport  Port=17
  line03_C3 : Inport  Port=18
  line03_dDisStart : Inport  Port=19
  line03_dDisEnd : Inport  Port=20
  line04_C0 : Inport  Port=21
  line04_C1 : Inport  Port=22
  line04_C2 : Inport  Port=23
  line04_C3 : Inport  Port=24
  line04_dDisStart : Inport  Port=25
  line04_dDisEnd : Inport  Port=26
  line05_C0 : Inport  Port=27
  line05_C1 : Inport  Port=28
  line05_C2 : Inport  Port=29
  line05_C3 : Inport  Port=30
  line05_dDisStart : Inport  Port=31
  line05_dDisEnd : Inport  Port=32
  line06_C0 : Inport  Port=33
  line06_C1 : Inport  Port=34
  line06_C2 : Inport  Port=35
  line06_C3 : Inport  Port=36
  line06_dDisStart : Inport  Port=37
  line06_dDisEnd : Inport  Port=38
  Action Port : ActionPort  ActionPortLabel=else
  Constant1 : Constant  Value=C_TOS_DefaultValueObjectToCenterLine_dy  OutDataTypeStr=single
      settings: AttributesFormatString=C_TOS_DefaultValueObjectToCenterLine_dy = 255
  Subtract : Sum  Inputs=+-
  Switch{,1..5} (6 alike) : Switch  Criteria=u2 ~= 0
  line01_DisJudge : Subsystem
  line01_dy : Subsystem
  line02_DisJudge : Subsystem
  line02_dy : Subsystem
  line03_DisJudge : Subsystem
  line03_dy : Subsystem
  line04_DisJudge : Subsystem
  line04_dy : Subsystem
  line05_DisJudge : Subsystem
  line05_dy : Subsystem
  line06_DisJudge : Subsystem
  line06_dy : Subsystem
  PP_ObjectToCenterLine_dy : Outport
  wires:
  line03_C0/1 -> line03_dy/2(line03_C0)
  line01_C3/1 -> line01_dy/5(line01_C3)
  line02_C1/1 -> line02_dy/3(line02_C1)
  line05_C2/1 -> line05_dy/4(line05_C2)
  line02_DisJudge/1(line02_DisJudge) -> Switch1/2
  line03_C3/1 -> line03_dy/5(line03_C3)
  [Object_DX] -> line05_dy/1(Object_DX)
  [Object_DX] -> line04_dy/1(Object_DX)
  Switch1/1 -> Switch/3
  line04_C2/1 -> line04_dy/4(line04_C2)
  line03_dDisEnd/1 -> line03_DisJudge/3(line03_dDisEnd)
  [Object_DX] -> line06_dy/1(Object_DX)
  line05_C3/1 -> line05_dy/5(line05_C3)
  Switch2/1 -> Switch1/3
  line02_C0/1 -> line02_dy/2(line02_C0)
  line02_C2/1 -> line02_dy/4(line02_C2)
  line05_dDisStart/1 -> line05_DisJudge/2(line05_dDisStart)
  line03_C2/1 -> line03_dy/4(line03_C2)
  line05_C1/1 -> line05_dy/3(line05_C1)
  line06_C2/1 -> line06_dy/4(line06_C2)
  line06_dy/1(line6_dy) -> Switch5/1
  [Object_DX] -> line02_DisJudge/1(Object_DX)
  line01_dy/1(line01_dy) -> Switch/1
  Object_DY/1 -> Subtract/1
  Switch4/1 -> Switch3/3
  line01_DisJudge/1(line01_DisJudge) -> Switch/2
  line06_dDisEnd/1 -> line06_DisJudge/3(line06_dDisEnd)
  line01_C2/1 -> line01_dy/4(line01_C2)
  line04_C3/1 -> line04_dy/5(line04_C3)
  [Object_DX] -> line02_dy/1(Object_DX)
  line04_C1/1 -> line04_dy/3(line04_C1)
  line04_DisJudge/1(line04_DisJudge) -> Switch3/2
  line02_C3/1 -> line02_dy/5(line02_C3)
  line04_dy/1(line04_dy) -> Switch3/1
  Switch3/1 -> Switch2/3
  line06_DisJudge/1(line06_DisJudge) -> Switch5/2
  line03_dy/1(line03_dy) -> Switch2/1
  line02_dy/1(line02_dy) -> Switch1/1
  line03_DisJudge/1(line03_DisJudge) -> Switch2/2
  line05_DisJudge/1(line05_DisJudge) -> Switch4/2
  Switch5/1 -> Switch4/3
  line06_C1/1 -> line06_dy/3(line06_C1)
  [Object_DX] -> line03_DisJudge/1(Object_DX)
  line01_dDisStart/1 -> line01_DisJudge/2(line01_dDisStart)
  line03_C1/1 -> line03_dy/3(line03_C1)
  line06_C0/1 -> line06_dy/2(line06_C0)
  line06_C3/1 -> line06_dy/5(line6_C3)
  line02_dDisStart/1 -> line02_DisJudge/2(line02_dDisStart)
  Switch/1 -> Subtract/2
  line03_dDisStart/1 -> line03_DisJudge/2(line03_dDisStart)
  Constant1/1 -> Switch5/3
  line04_dDisStart/1 -> line04_DisJudge/2(line04_dDisStart)
  line04_C0/1 -> line04_dy/2(line04_C0)
  line01_C1/1 -> line01_dy/3(line01_C1)
  [Object_DX] -> line03_dy/1(Object_DX)
  line01_dDisEnd/1 -> line01_DisJudge/3(line01_dDisEnd)
  [Object_DX] -> line01_DisJudge/1(Object_DX)
  line05_dy/1(line05_dy) -> Switch4/1
  [Object_DX] -> line04_DisJudge/1(Object_DX)
  [Object_DX] -> line05_DisJudge/1(Object_DX)
  line01_C0/1 -> line01_dy/2(line01_C0)
  line06_dDisStart/1 -> line06_DisJudge/2(line06_dDisStart)
  line04_dDisEnd/1 -> line04_DisJudge/3(line04_dDisEnd)
  line05_C0/1 -> line05_dy/2(line05_C0)
  line05_dDisEnd/1 -> line05_DisJudge/3(line05_dDisEnd)
  [Object_DX] -> line06_DisJudge/1(Object_DX)
  line02_dDisEnd/1 -> line02_DisJudge/3(line02_dDisEnd)
  Object_DX/1 -> [Object_DX], line01_dy/1(Object_DX)
  Subtract/1 -> PP_ObjectToCenterLine_dy/1

== system PubIfDecisionTOS_MDL/TOS_20201112/TOS_2012080320/PP1128/AAT-AdditionalAttributes/PP_ObjectToCenterLine_dy/PP_ObjectToCenterLine_vyc/PP_ObjectToCenterLine_vyc_Filt/ObjectToCenterLine_vyc ==
  ObjectID_Filt_K1 : Inport
  PP_ObjectToCenterLine_vyc_Filt_K1 : Inport  Port=2  OutDataTypeStr=single
  PP_ObjectToCenterLine_vyc : Inport  Port=3  OutDataTypeStr=single  Partition=on  PartitionDimension=1  PartitionWidth=1  PartitionOffset=0
  TOS_OFMObjValid_Flag : Inport  Port=4  OutDataTypeStr=uint8  Partition=on  PartitionDimension=1  PartitionWidth=1  PartitionOffset=0
  Object_ID : Inport  Port=5  OutDataTypeStr=uint8  Partition=on  PartitionDimension=1  PartitionWidth=1  PartitionOffset=0
  Object_Age : Inport  Port=6  Partition=on  PartitionDimension=1  PartitionWidth=1  PartitionOffset=0
  Compare To Constant : simulink/Logic and Bit Operations/Compare To Constant  relop===  const=C_TOS_OFMObjIDInvilad_Val  OutDataTypeStr=boolean
      settings: AttributesFormatString=C_TOS_OFMObjIDInvilad_Val = 0
  For Each : ForEach  DisableCoverage=on
  If : If  IfExpression=u1 ~= 0
  Merge : Merge
  Merge1 : Merge
  ObjectToCenterLine_vyc_Filt : Subsystem
  ObjectToCenterLine_vyc_FiltDefault : Subsystem  TreatAsAtomicUnit=on
  Obj_ID : Outport  ConcatenationDimension=1
  PP_ObjectToCenterLine_vyc_Filt : Outport  Port=2  OutDataTypeStr=single  ConcatenationDimension=1
  wires:
  [TOS_OFMObjValid_Flag] -> ObjectToCenterLine_vyc_Filt/6(TOS_OFMObjValid_Flag)
  TOS_OFMObjValid_Flag/1 -> Compare To Constant/1, [TOS_OFMObjValid_Flag]
  Object_Age/1 -> ObjectToCenterLine_vyc_Filt/5(Object_Age)
  Merge/1 -> Obj_ID/1
  Merge1/1 -> PP_ObjectToCenterLine_vyc_Filt/1
  ObjectToCenterLine_vyc_FiltDefault/2(ObjectToCenterLine_dy_Filt) -> Merge1/1
  ObjectToCenterLine_vyc_FiltDefault/1(Obj_ID) -> Merge/1
  ObjectToCenterLine_vyc_Filt/2(PP_ObjectToCenterLine_vyc_Filt) -> Merge1/2
  ObjectToCenterLine_vyc_Filt/1(Obj_ID) -> Merge/2
  PP_ObjectToCenterLine_vyc/1 -> ObjectToCenterLine_vyc_Filt/3(PP_ObjectToCenterLine_vyc)
  PP_ObjectToCenterLine_vyc_Filt_K1/1 -> ObjectToCenterLine_vyc_Filt/2(PP_ObjectToCenterLine_vyc_Filt_K1)
  ObjectID_Filt_K1/1 -> ObjectToCenterLine_vyc_Filt/1(ObjectID_Filt_K1)
  Compare To Constant/1 -> If/1
  Object_ID/1 -> ObjectToCenterLine_vyc_Filt/4(Object_ID)
  If/1 -> ObjectToCenterLine_vyc_FiltDefault/Action
  If/2 -> ObjectToCenterLine_vyc_Filt/Action
